simulink model "zetimerpot"  (R2018a)
settings: Solver=FixedStepDiscrete  StartTime=0.0  StopTime=50  FixedStep=1e-4  RelTol=1e-3  EnableMultiTasking=on
InitFcn:
  | mbd_pnt_consistency_checks(bdroot(gcs));
undefined symbols (not defined in the file): AN, B, B14, C10, J, P9, PCR, R5, T12, T13
libraries: mbd_pnt_ec_toolbox x6, dspswit3 x1
Description:
  | This model shows how to measure the PWM signal period with eTimer
  | 
  | The FlexPWM module 0, submodule 0, is configured to generated a PWM waveform
  | on A10 and A11 pins (J1.5 and J1.7). The frequency is changing @5sec between
  | 1000Hz and 10000Hz
  | 
  | The eTimer is configured to read the signal from A0 (J5.1)
  | 
  | Connect a wire between any of J1.5/J1.7 and J5.1 to have meaningfull data.
settings Model: Creator=vkostrov  LastModifiedBy=oolonthegreat
settings DataIOCC: ExternalInput=off  InitialState=off  LimitDataPoints=on  SaveFormat=Array  SignalLoggingSaveFormat=ModelDataLogs  SaveOutput=off  SignalLogging=off  SaveTime=off
settings OptimizationCC: DefaultParameterBehavior=Inlined  ExpressionDepthLimit=2147483647  LifeSpan=1
settings DebuggingCC: UnderspecifiedInitializationDetection=Classic  MergeDetectMultiDrivingBlocksExec=none  SolverPrmCheckMsg=warning  InheritedTsInSrcMsg=none  SingleTaskRateTransMsg=error  FcnCallInpInsideContextMsg=warning  UnconnectedInputMsg=error  UnconnectedOutputMsg=error  UnconnectedLineMsg=error  AllowSymbolicDim=off  UnknownTsInhSupMsg=error  StateNameClashWarn=warning  SFUnexpectedBacktrackingDiag=warning  SFNoUnconditionalDefaultTransitionDiag=warning  SFExecutionAtInitializationDiag=none
settings HardwareCC: ProdBitPerPointer=32  ProdBitPerSizeT=32  ProdBitPerPtrDiffT=32  ProdLargestAtomicInteger=Long  ProdLargestAtomicFloat=Double  ProdEndianess=BigEndian  ProdWordSize=32  ProdHWDeviceType=Motorola PowerPC
settings ModelReferenceCC: PropagateSignalLabelsOutOfModel=off
settings SFSimCC: MATLABDynamicMemAlloc=off
settings RTWCC: SystemTargetFile=mbd_pnt.tlc  MakeCommand=mbd_pnt_make_rtw COPY_MDLREF_INCLUDES=0  TemplateMakefile=mbd_pnt.tmf  PostCodeGenCommand=mbd_pnt_analyzegencode(buildInfo)  Description=Model Based Design Toolbox MPC574xP Code Generation Target
settings CodeAppCC: IgnoreCustomStorageClasses=off  CustomSymbolStrType=$N$R$M  StateflowObjectComments=on  InternalIdentifier=Classic
settings STFCustomTargetCC: CombineOutputUpdateFcns=on  SuppressErrorStatus=on  ERTCustomFileBanners=on  SupportContinuousTime=off  SupportNonInlinedSFcns=off  RemoveResetFunc=on  MATLABClassNameForMDSCustomization=Simulink.SoftwareTarget.ERTCustomization  GRTInterface=off  SystemTargetFile=mbd_pnt.tlc
settings ERTTargetCC: MultiwordLength=2048  ParMdlRefBuildCompliant=off  CompOptLevelCompliant=off  ConcurrentExecutionCompliant=off  SuppressErrorStatus=on  ModelStepFunctionPrototypeControlCompliant=off  CPPClassGenCompliant=off  UseToolchainInfoCompliant=off  ExtModeMexFile=noextcomm  InlinedParameterPlacement=NonHierarchical  ERTCustomFileTemplate=example_file_process.tlc  ConvertIfToSwitch=off  SuppressUnreachableDefaultCases=off
settings ConfigComp: CovMetricSettings=dw  CovHtmlReporting=on  CovSaveCumulativeToWorkspaceVar=on  CovSaveSingleToWorkspaceVar=on  CovExternalEMLEnable=off

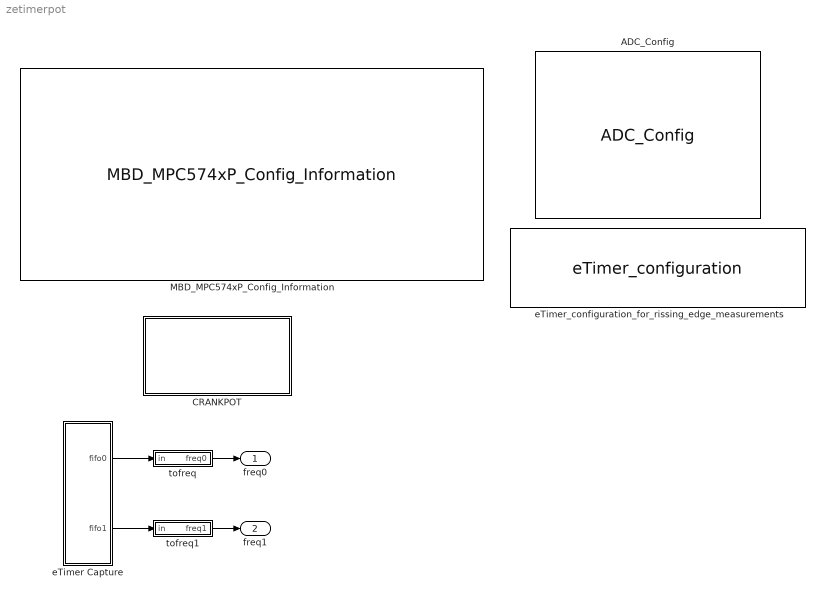
== system zetimerpot ==
  ADC_Config : mbd_pnt_ec_toolbox/MPC574xP/Motor Control Blocks/ADC_Config  adc_unit=1  adc_ctu=off  adc_owr=on  adc_wls=0: Left  adc_clk=on  adc_ack=on  adc_edglev=0: Edge  adc_trgen=off  adc_edge=off  adc_ctr0_samp=22  adc_ctr1_samp=11  adc_pscr_preval0=00: AGND_3V  adc_pscr_preconv=off  adc_calbist_admode=110: 12-bit operating mode (high accuracy)  adc_calbist_tsamp=00: 22 cycles of ADC clk  adc_calbist_nrsmpl=01: 32 samples  adc_calbist_avgen=on
      settings: SourceProductName=Model Based Design Toolbox for MPC574xP
  CRANKPOT : Subsystem
  MBD_MPC574xP_Config_Information : mbd_pnt_ec_toolbox/MPC574xP/MBD_MPC574xP_Config_Information  disp_str=|  config_params=[]
      | System Clock : 200 MHz
      | Target : MPC5744P
      | Package : 144LQFP
      | XTAL Freq : 40 MHz
      | Compiler : S32 Design Studio
      | Target Type : FLASH
      | Global Interrupt Priority : 8
      | System Tick Interrupt Priority : 12
      | Freemaster : Serial1 (115200 Kbits)
      | Download Code after build : (COM5,115200)
      settings: SourceProductName=Model Based Design Toolbox for MPC574xP
  eTimer Capture : Subsystem
  eTimer_configuration_for_rissing_edge_measurements : mbd_pnt_ec_toolbox/MPC574xP/Motor Control Blocks/eTimer_configuration  SubModule=0  TimerChan=0  subMod=0  channel=0  CountMode=001 - Count rising edges of primary source  CNTMODE=1  CountOnce=0 - Count repeatedly  ONCE=0  CountLength=0 - Continue counting to roll over  LENGTH=0  CountDirection=0 - Count up  DIR=0  OutputEnable=0 - The external pin is configured as an input  OEN=0  CoChanInit=00 - Other channels cannot force re-initialization of this channel  COINIT=0  StopAction=0 - Output enable is unaffected by stop mode  STPEN=0  ReloadOnCapt=01 - Reload the counter on a capture 1 event  ROC=1  PrimarySource=11111 - IP Bus clock divide by 128 prescaler  PRISRC=31  PrimSrcPol=0 - True polarity  PIPS=0  SecondarySource=00000 - Counter #0 input pin  SECSRC=0  SecSrcPol=0 - True polarity  SIPS=0  FILT_CNT=0  FILT_PER=0  FILT=0  OutputMode=0000 - Software controlled  OUTMODE=0  OutputPol=0 - True polarity  OPS=0  MasterMode=0 - Disable broadcast of this channel output  MSTR=0  ForcedOutVal=0  VAL=0  CoForce=0 - Other channels cannot force this channel output  COFRC=0  CompLoad1=000 - COMP1 is never preload  CLC1=0  CompLoad2=000 - COMP2 is never preload  CLC2=0  CompareMode="00 - COMP1 and COMP2  are used when the counter is counting up"  CMPMODE=0  CaptMode1=10 - Capture rising edges  CPT1MODE=2  CaptMode2=00 - Capture disabled  CPT2MODE=0  OneShCaptMode=0 - Free running mode is selected  ONESHOT=0  CaptFIFO=0  CFWM=0  CNTRinit=0  COMP1init=0  COMP2init=0  mod0ch0pin="0     : A0   :  [73]   : [86]   : [P12]  input/output"  mod0ch1pin=None  mod0ch2pin=None  mod0ch3pin=None  mod0ch4pin=None  mod0ch5pin=None  mod1ch0pin=None  mod1ch1pin=None  mod1ch2pin=None  mod1ch3pin=None  mod1ch4pin=None  mod1ch5pin=None  mod2ch0pin=None  mod2ch1pin=None  mod2ch2pin=None  mod2ch3pin=None  mod2ch4pin=None  mod2ch5pin=None  pcrNum0=0  pcrNum1=255  pcrNum2=255  pcrNum3=255  pcrNum4=255  pcrNum5=255  TCFIE=off  TCF1IE=off  TCF2IE=off  TOFIE=off  IELFIE=off  IEHFIE=off  ICF1IE=off  ICF2IE=off  INTDMA=0
      settings: SourceProductName=Model Based Design Toolbox for MPC574xP
  tofreq : Subsystem
  tofreq1 : Subsystem
  freq0 : Outport
  freq1 : Outport  Port=2
  wires:
  eTimer Capture/1(fifo0) -> tofreq/1(in)
  eTimer Capture/2(fifo1) -> tofreq1/1(in)
  tofreq1/1(freq1) -> freq1/1
  tofreq/1(freq0) -> freq0/1

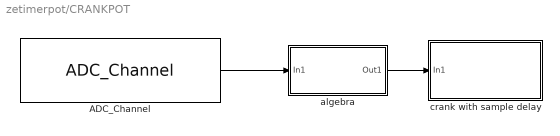
== system zetimerpot/CRANKPOT ==
  ADC_Channel : mbd_pnt_ec_toolbox/MPC574xP/Motor Control Blocks/ADC_Channel  adc_unit=1  adc_chan0=PCR[23] : B[7] : 43 : 51 : R5 : AN[0]  adc_chan1=PCR[76] : E[12] : 67 : 78 : T12 : AN[6]  adc_chan2=PCR[150] : J[6] : [---] : 65 : P9 : AN[1]  adc_chan3=PCR[64] : E[0] : 68 : 79 : T13 : AN[4]  simulate=off  interrupt=off  adc_mode=Normal  adc_presample=off  pcrNum=76
      settings: SourceProductName=Model Based Design Toolbox for MPC574xP
  algebra : Subsystem
  crank with sample delay : Subsystem
  wires:
  ADC_Channel/1 -> algebra/1(In1)
  algebra/1(Out1) -> crank with sample delay/1(In1)

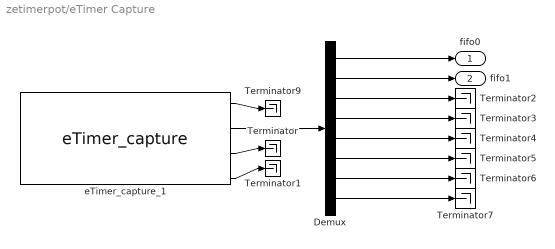
== system zetimerpot/eTimer Capture ==
  Demux : Demux  Outputs=8
  Terminator{,1..7,9} (9 alike) : Terminator
  eTimer_capture_1 : mbd_pnt_ec_toolbox/MPC574xP/Motor Control Blocks/eTimer_capture  SubModule=0  Timerchan=0  subMod=0  channel=0
      settings: SourceProductName=Model Based Design Toolbox for MPC574xP
  fifo0 : Outport
  fifo1 : Outport  Port=2
  wires:
  Demux/4 -> Terminator3/1
  eTimer_capture_1/3 -> Terminator/1
  eTimer_capture_1/2 -> Demux/1
  Demux/8 -> Terminator7/1
  Demux/7 -> Terminator6/1
  Demux/5 -> Terminator4/1
  Demux/3 -> Terminator2/1
  eTimer_capture_1/4 -> Terminator1/1
  Demux/6 -> Terminator5/1
  Demux/2 -> fifo1/1
  eTimer_capture_1/1 -> Terminator9/1
  Demux/1 -> fifo0/1

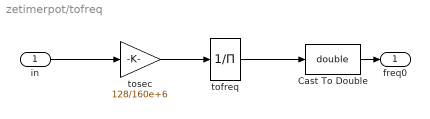
== system zetimerpot/tofreq ==
  in : Inport
  Cast To Double : DataTypeConversion  OutDataTypeStr=double
  tofreq : Product  Inputs=/  OutDataTypeStr=uint16  RndMeth=Ceiling
  tosec : Gain  Gain=128/160e+6  OutDataTypeStr=double  RndMeth=Ceiling
  freq0 : Outport
  wires:
  tosec/1 -> tofreq/1
  tofreq/1 -> Cast To Double/1
  in/1 -> tosec/1
  Cast To Double/1 -> freq0/1

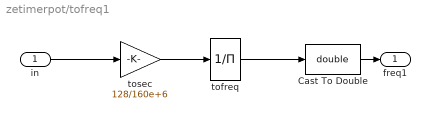
== system zetimerpot/tofreq1 ==
  in : Inport
  Cast To Double : DataTypeConversion  OutDataTypeStr=double
  tofreq : Product  Inputs=/  OutDataTypeStr=uint16  RndMeth=Ceiling
  tosec : Gain  Gain=128/160e+6  OutDataTypeStr=double  RndMeth=Ceiling
  freq1 : Outport
  wires:
  tosec/1 -> tofreq/1
  tofreq/1 -> Cast To Double/1
  in/1 -> tosec/1
  Cast To Double/1 -> freq1/1

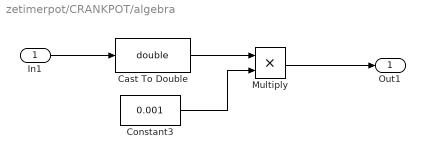
== system zetimerpot/CRANKPOT/algebra ==
  In1 : Inport
  Cast To Double : DataTypeConversion  OutDataTypeStr=double
  Constant3 : Constant  Value=0.001
  Multiply : Product
  Out1 : Outport
  wires:
  Constant3/1 -> Multiply/2
  Cast To Double/1 -> Multiply/1
  In1/1 -> Cast To Double/1
  Multiply/1 -> Out1/1

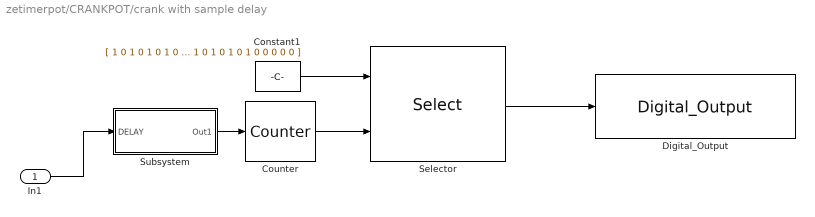
== system zetimerpot/CRANKPOT/crank with sample delay ==
  In1 : Inport
  Constant1 : Constant  Value=[ 1 0 1 0 1 0 1 0 1 0 1 0 1 0 1 0 1 0 1 0 1 0 1 0 1 0 1 0 1 0 1 0 1 0 1 0 0 0 0 0 1 0 1 0 1 0 1 0 1 0 1 0 1 0 1 0 1 0 1 0 1 0 1 0 1 0 1 0 1 0 1 0 1 0 1 0 0 0 0 0 1 0 1 0 1 0 1 0 1 0 1 0 1 0 1 0 1 0 1 0 1 0 1 0 1 0 1 0 1 0 1 0 1 0 1 0 0 0 0 0 1 0 1 0 1 0 1 0 1 0 1 0 1 0 1 0 1 0 1 0 1 0 1 0 1 0 1 0 1 0 1 0 1 0 1 0 0 0 0 0 1 0 1 0 1 0 1 0 1 0 1 0 1 0 1 0 1 0 1 0 1 0 1 0 1 0 1 0 1 0 1 0 1 0 1 0 0 0 0 0 1 0 1 0 1 0 1 0 1 0 1 0 1 0 1 0 1 0 1 0 1 0 1 0 1 0 1 0 1 0 1 0 1 0 1 0 0 0 0 0 ]  OutDataTypeStr=boolean
  Counter : dspswit3/Counter  Direction=Up  CountEvent=Rising edge  CounterSize=User defined  MaxCount=239  InitialCount=0  Output=Count  HitValue=32  ResetInput=off  SamplesPerFrame=1  Ts=1  CntDtype=double  HitDtype=Logical
  Digital_Output : mbd_pnt_ec_toolbox/MPC574xP/Peripheral Interface Blocks/Digital_Output  gpio_outputs="42   : C10 :  [111] : [136] : [B14]"  pinNum=[111]  pcrNum=42
      settings: SourceProductName=Model Based Design Toolbox for MPC574xP
  Selector : Selector  IndexMode=Zero-based  InputPortWidth=240  IndexOptions=Index vector (port)  Indices=[1 3]  OutputSizes=1
  Subsystem : Subsystem
  wires:
  Subsystem/1(Out1) -> Counter/1
  Selector/1 -> Digital_Output/1
  Counter/1 -> Selector/2
  In1/1 -> Subsystem/1(DELAY)
  Constant1/1 -> Selector/1

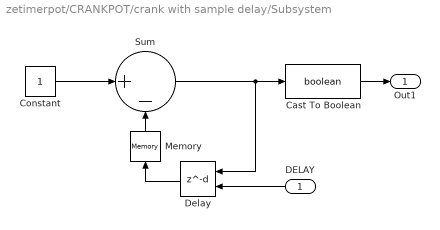
== system zetimerpot/CRANKPOT/crank with sample delay/Subsystem ==
  DELAY : Inport
  Cast To Boolean : DataTypeConversion  OutDataTypeStr=boolean
  Constant : Constant  OutDataTypeStr=double
  Delay : Delay  DelayLengthSource=Input port
      settings: InputPortMap=u0,p1
  Memory : Memory
  Sum : Sum  Inputs=|+-  OutDataTypeStr=double
  Out1 : Outport
  wires:
  Constant/1 -> Sum/1
  Sum/1 -> Cast To Boolean/1, Delay/1
  Delay/1 -> Memory/1
  DELAY/1 -> Delay/2
  Memory/1 -> Sum/2
  Cast To Boolean/1 -> Out1/1
